simulink model "siavash_walking"  (R2014b)
settings: Solver=FixedStepDiscrete  StartTime=0.0  StopTime=inf  FixedStep=sample_time  RelTol=1e-3
StartFcn:
  | tg.sampletime = correctedSampleTime;
libraries: slrtlib x1
settings Model: SimulationMode=external  BufferReuse=off  Creator=wmartin  LastModifiedBy=robots
settings SolverCC: EnableConcurrentExecution=on
settings DataIOCC: LimitDataPoints=off  MaxDataPoints=1e7  SaveFormat=StructureWithTime  SignalLogging=off  DSMLogging=off
settings OptimizationCC: BlockReduction=off  OptimizeBlockIOStorage=off  BufferReuse=off  GlobalBufferReuse=off  ExpressionFolding=off  ExpressionDepthLimit=2147483647  LocalBlockOutputs=off  SimCompilerOptimization=On
settings DebuggingCC: UnderspecifiedInitializationDetection=Classic  MergeDetectMultiDrivingBlocksExec=none  StateNameClashWarn=warning
settings HardwareCC: ProdIntDivRoundTo=Zero  ProdEndianess=LittleEndian  ProdLongLongMode=on  ProdHWDeviceType=Generic->32-bit x86 compatible
settings ModelReferenceCC: UpdateModelReferenceTargets=IfOutOfDate  ModelReferenceNumInstancesAllowed=Single  ModelReferenceMinAlgLoopOccurrences=on
settings RTWCC: SystemTargetFile=slrt.tlc  TemplateMakefile=slrt_default_tmf  Description=Simulink Real-Time  RTWVerbose=off  ProcessScript=slrt_make_rtw_hook  RTWCompilerOptimization=On
settings CodeAppCC: MaxIdLength=256
settings SimulinkRealTimeCC: GeneratePreprocessorConditionals=Disable all  EnableShiftOperators=on  RL32LogBufSizeModifier=1e8

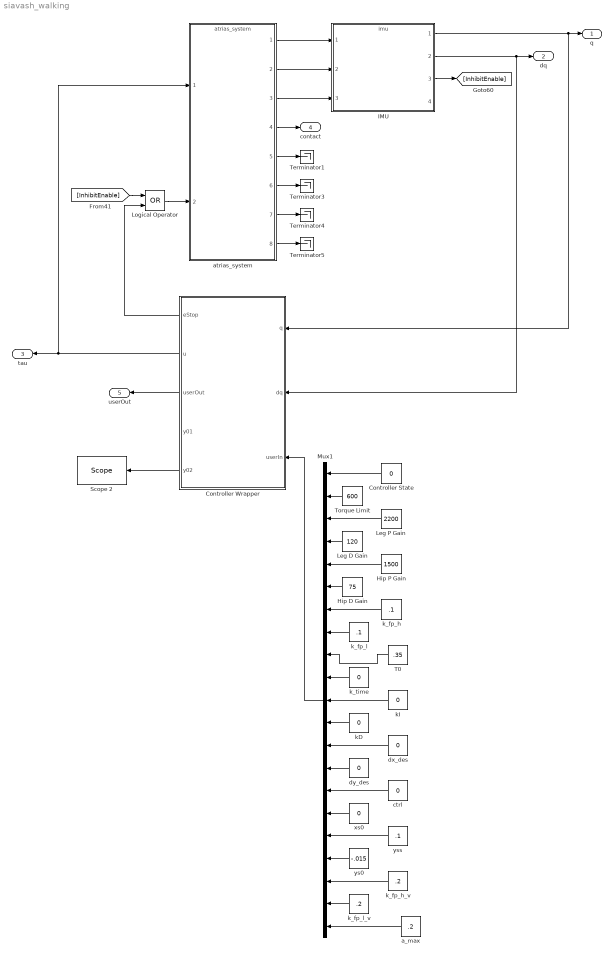
== system siavash_walking ==
  Controller State : Constant  Value=0
  Controller Wrapper : MATLAB Function  TreatAsAtomicUnit=on
  Hip D Gain : Constant  Value=75
  Hip P Gain : Constant  Value=1500
  IMU : ModelReference  ModelNameDialog=imu  SimulationMode=Normal  ModelReferenceVersion=1.2451  CopyOfModelName=imu  DefaultDataLogging=on
  Leg D Gain : Constant  Value=120
  Leg P Gain : Constant  Value=2200
  Logical Operator : Logic  Operator=OR  AllPortsSameDT=off  OutDataTypeStr=boolean
  Mux1 : Mux  Inputs=21
  Scope 2 : slrtlib/Displays and Logging/Scope   scopeno=1  scopetype=Target  autostart=on  viewmode=Graphical sliding  formatstr='%15.6f'  grid=on  ylimits=[0,0]  nosamples=3000  noprepostsamples=0  interleave=1  triggermode=FreeRun  triggersignal=1  trigsignalfromport=off  triggerlevel=0.0  triggerslope=Either  triggerscope=1  triggersample=0  filename=data.dat  mode=Lazy  writesize=512  autorestart=off  dynamicfilemode=off  maxwritefilesize=512*1024^2
  T0 : Constant  Value=.35
  Terminator{1,3..5} (4 alike) : Terminator
  Torque Limit : Constant  Value=600
  a_max : Constant  Value=.2
  atrias_system : ModelReference  ModelNameDialog=atrias_system  SimulationMode=Normal  ModelReferenceVersion=1.2603  CopyOfModelName=atrias_system  DefaultDataLogging=on
  ctrl : Constant  Value=0
  dx_des : Constant  Value=0
  dy_des : Constant  Value=0
  kD : Constant  Value=0
  kI : Constant  Value=0
  k_fp_h : Constant  Value=.1
  k_fp_h_v : Constant  Value=.2
  "k_fp_l " : Constant  Value=.1
  k_fp_l_v : Constant  Value=.2
  k_time : Constant  Value=0
  xs0 : Constant  Value=0
  ys0 : Constant  Value=-.015
  yss : Constant  Value=.1
  q : Outport
  dq : Outport  Port=2
  tau : Outport  Port=3
  contact : Outport  Port=4
  userOut : Outport  Port=5
  wires:
  atrias_system/4 -> contact/1
  atrias_system/5 -> Terminator1/1
  atrias_system/7 -> Terminator4/1
  atrias_system/6 -> Terminator3/1
  atrias_system/8 -> Terminator5/1
  Controller Wrapper/2(u) -> atrias_system/1, tau/1
  Mux1/1 -> Controller Wrapper/3(userIn)
  Controller State/1 -> Mux1/1
  Torque Limit/1 -> Mux1/2
  Leg P Gain/1 -> Mux1/3
  Leg D Gain/1 -> Mux1/4
  Hip P Gain/1 -> Mux1/5
  Hip D Gain/1 -> Mux1/6
  IMU/3 -> [InhibitEnable]
  IMU/1 -> Controller Wrapper/1(q), q/1
  IMU/2 -> Controller Wrapper/2(dq), dq/1
  atrias_system/1 -> IMU/1
  atrias_system/2 -> IMU/2
  atrias_system/3 -> IMU/3
  [InhibitEnable] -> Logical Operator/1
  Logical Operator/1 -> atrias_system/2
  Controller Wrapper/1(eStop) -> Logical Operator/2
  Controller Wrapper/5(y02) -> Scope 2/1
  k_fp_h/1 -> Mux1/7
  "k_fp_l "/1 -> Mux1/8
  T0/1 -> Mux1/9
  k_time/1 -> Mux1/10
  kI/1 -> Mux1/11
  kD/1 -> Mux1/12
  dx_des/1 -> Mux1/13
  dy_des/1 -> Mux1/14
  Controller Wrapper/3(userOut) -> userOut/1
  ctrl/1 -> Mux1/15
  xs0/1 -> Mux1/16
  yss/1 -> Mux1/17
  ys0/1 -> Mux1/18
  k_fp_h_v/1 -> Mux1/19
  k_fp_l_v/1 -> Mux1/20
  a_max/1 -> Mux1/21

== matlab function siavash_walking/Controller Wrapper ==
  data: eStop output; q input; u output; dq input; userIn input; userOut output; y01 output; y02 output
function [eStop, u, userOut, y01, y02] = wrapper(q, dq, userIn)
%WRAPPER Controller wrapper.
%
% Notes:
% 	- State indexes (q and qdot)
%       (rBl rBm rAl rAm lBl lBm lAl lAm rHm lHm bR bY bP) 
%   - Input indexes (u)
%       (rB rA rH lB lA lH)
    
    % CMU --> OSU coordinates
%     q(9) = -q(9); dq(9) = -dq(9);
    
    % Replace boom data with IMU data here
    
    % Actual controller function
    [eStop, u, userOut, y01, y02] = controller3Dwalking5(q, dq, userIn);
        
    % OSU --> CMU coordinates
%     u = -u; u(3) = -u(3);
end % wrapper
